simulink subsystem "Ctrl_Reg_1"  (R2025b)
settings: Solver=VariableStepAuto  StartTime=0.0  StopTime=10.0  RelTol=1e-3
values from neighbouring files (symbols this model uses):
  ctrl_reg1 = 0x02    [PMSM_to_BLDC_FOC.m]
  reg_ctrl_1 = ( bitshift(21,6) + bitshift(1,4) + bitshift(0,3) + bitshift(0,2) + bitshift(0,0))    [PMSM_to_BLDC_FOC.m]
  write_reg = 0    [PMSM_to_BLDC_FOC.m]
libraries: hdlsllib x2, simulink x2, stm32blockslib x1
settings Model: STM32="{\"SPIControllerTransmit\":[{\"ID\":\"Ctrl_Reg_1:1032\"},{\"ID\":\"Ctrl_Reg_1:1184\"}]}"  Creator=Surinova  LastModifiedBy=Surinova

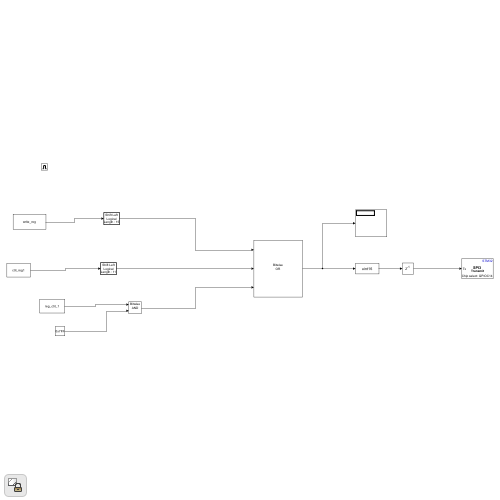
[thumbnail: Simulink's stored preview of the top-level diagram]
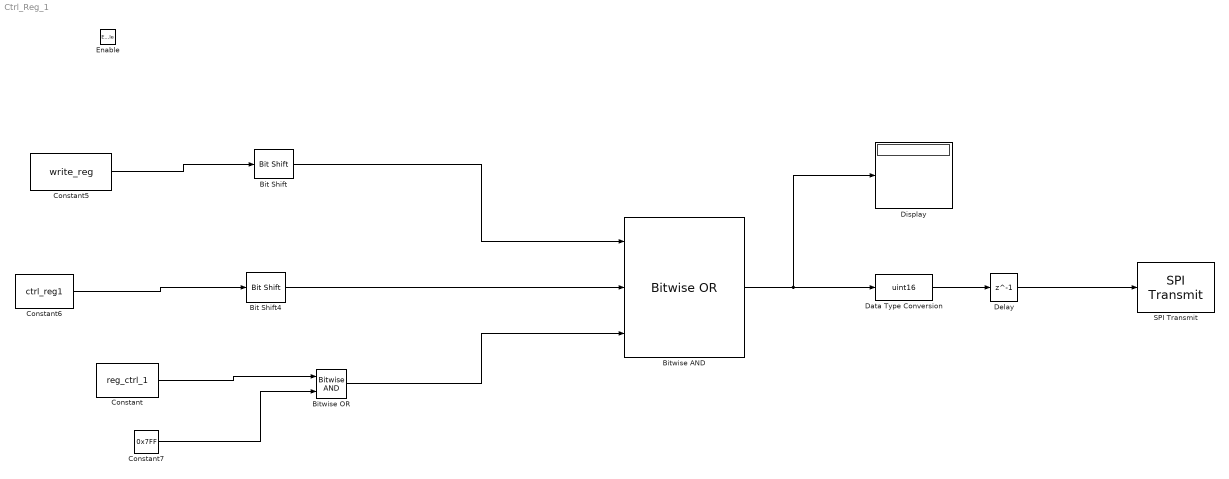
== system Ctrl_Reg_1 ==
  Enable : EnablePort  StatesWhenEnabling=reset  PropagateVarSize=During execution
  Bit Shift : hdlsllib/Logic and Bit Operations/Bit Shift  mode=Shift Left Logical  N=15
  Bit Shift4 : hdlsllib/Logic and Bit Operations/Bit Shift  mode=Shift Left Logical  N=11
  Bitwise AND : simulink/Logic and Bit Operations/Bitwise Operator  logicop=OR  UseBitMask=off  NumInputPorts=3  BitMask=bin2dec('11011001')  BitMaskRealWorld=Stored Integer
      settings: LibrarySourceBlock=|
      | simulink/Quick Insert/Logic and Bit
      | Operations/Bitwise AND
  Bitwise OR : simulink/Logic and Bit Operations/Bitwise Operator  logicop=AND  UseBitMask=off  NumInputPorts=2  BitMask=bin2dec('11011001')  BitMaskRealWorld=Stored Integer
      settings: LibrarySourceBlock=|
      | simulink/Quick Insert/Logic and Bit
      | Operations/Bitwise OR
  Constant : Constant  Value=reg_ctrl_1  OutDataTypeStr=uint16
  Constant5 : Constant  Value=write_reg  OutDataTypeStr=uint16
  Constant6 : Constant  Value=ctrl_reg1  OutDataTypeStr=uint16
  Constant7 : Constant  Value=0x7FF  OutDataTypeStr=uint16
  Data Type Conversion : DataTypeConversion  OutDataTypeStr=uint16  SaturateOnIntegerOverflow=off  RndMeth=Floor
  Delay : Delay  DelayLength=1  InputProcessing=Columns as channels (frame based)  SampleTime=1
  Display : Display
      settings: Format=hex (Stored Integer)
  SPI Transmit : stm32blockslib/SPI Transmit  SPIModuleSelect=SPI3  ClockPolarity=Low  ClockPhase=2 Edge  SPIModule=uint32(0)  Mode=Master  BusSpeed=uint32(1000000)  FirstBitToTransfer=Most significant bit (MSB)  ClockMode=0  BlockFunction=Write  EnableRegisterAddress=on  RegisterAddress=0  OutputDataType=uint8  OutputDataLength=1  OutputStatus=off  BlockingMode=on  Timeout=0.01  DataBits=16  UseCustomSSPin=Explicit GPIO calls  ActiveLowSSPin=Active low  Port_Select=GPIOC  Pin=14
      settings: LibrarySourceBlock=stm32f4xxblockslib/SPI Transmit
  wires:
  Bit Shift/1 -> Bitwise AND/1
  Bit Shift4/1 -> Bitwise AND/2
  Constant7/1 -> Bitwise OR/2
  Bitwise AND/1 -> Data Type Conversion/1, Display/1
  Bitwise OR/1 -> Bitwise AND/3
  Constant5/1 -> Bit Shift/1
  Constant6/1 -> Bit Shift4/1
  Constant/1 -> Bitwise OR/1
  Data Type Conversion/1 -> Delay/1
  Delay/1 -> SPI Transmit/1
